simulink model "simulink_test"  (R2018a)
settings: Solver=FixedStepAuto  StartTime=0.0  StopTime=5  FixedStep=1  RelTol=1e-3
undefined symbols (not defined in the file): init, stop
settings Model: Creator=root  LastModifiedBy=root

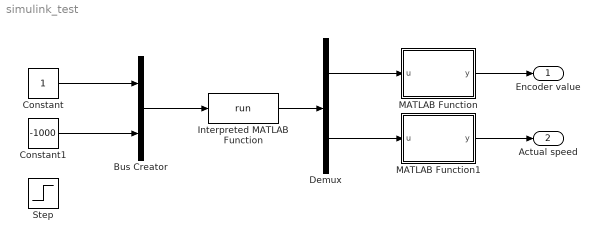
== system simulink_test ==
  Bus Creator : BusCreator  Inputs=2
  Constant : Constant
  Constant1 : Constant  Value=-1000
  Demux : Demux  Outputs=2
  Interpreted MATLAB Function : MATLABFcn  StartFcn=init([1])  StopFcn=stop([1])  MATLABFcn=run
  MATLAB Function : MATLAB Function  TreatAsAtomicUnit=on
  MATLAB Function1 : MATLAB Function  TreatAsAtomicUnit=on
  Step : Step  Time=5  Before=1000  After=1500  SampleTime=1
  Encoder value : Outport
  Actual speed : Outport  Port=2
  wires:
  Constant/1 -> Bus Creator/1
  Bus Creator/1 -> Interpreted MATLAB Function/1
  Constant1/1 -> Bus Creator/2
  Interpreted MATLAB Function/1 -> Demux/1
  Demux/1 -> MATLAB Function/1(u)
  MATLAB Function/1(y) -> Encoder value/1
  Demux/2 -> MATLAB Function1/1(u)
  MATLAB Function1/1(y) -> Actual speed/1

== matlab function simulink_test/MATLAB Function1 ==
  data: u input; y output
function y = fcn(u)
if (u > 4000000000)
    a = dec2bin(u - 1, 32);
    k = 32;
    for k = 1:32
        if a(k) == '0'
            a(k) = '1';
        else
            a(k) = '0';
        end
    end
    y = bin2dec(a)*(-1);
else
    y = u;
end

== matlab function simulink_test/MATLAB Function ==
  data: u input; y output
function y = fcn(u)
if (u > 4290000000)
    a = dec2bin(u - 1, 32);
    k = 32;
    for k = 1:32
        if a(k) == '0'
            a(k) = '1';
        else
            a(k) = '0';
        end
    end
    y = bin2dec(a)*(-1);
else
    y = u;
end
